simulink model "Progressive_Scan_Implementation_5x5_C"  (R2023a)
settings: Solver=VariableStepAuto  StartTime=0.0  StopTime=5  RelTol=1e-3
InitFcn:
  | Sampling_Time = 0.02;
  | 
  | % Find Controller
  | A_T= 3.6174;
  | tau = 1.2889;
  | Ts = Sampling_Time;
  | Kt = A_T * (1-exp(-Ts/tau));
  | poles = [-0.9180   -0.7439]; % 2x2
  | poles = [-0.5844   -0.9007]; % more aggressive
  | poles = [-0.7161   -0.8]; % 0.02 Ts aggro
  | poles = [-0.6161   -0.7]; % 0.02 Ts aggro
  | a1 = (poles(1)+poles(2)+1+exp(-Ts/tau))/Kt;
  | a0 = (poles(1)*poles(2)-exp(-Ts/tau))/Kt;
  | a1 = a1(1);
  | a0 = a0(1);
StopFcn:
  | datloc = out.varout{1}.Values;
  | 
  | t = datloc.Time;
  | T = datloc.Data;
  | writematrix([t T], "temp_out.csv");
  | cu = out.cuout{1}.Values;
  | writematrix([cu.Time cu.Data], "temp_control.csv");
settings Model: Creator=wangj  LastModifiedBy=wangj

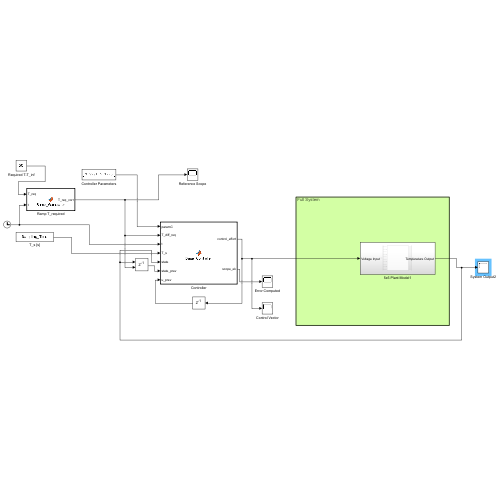
[thumbnail: Simulink's stored preview of the top-level diagram]
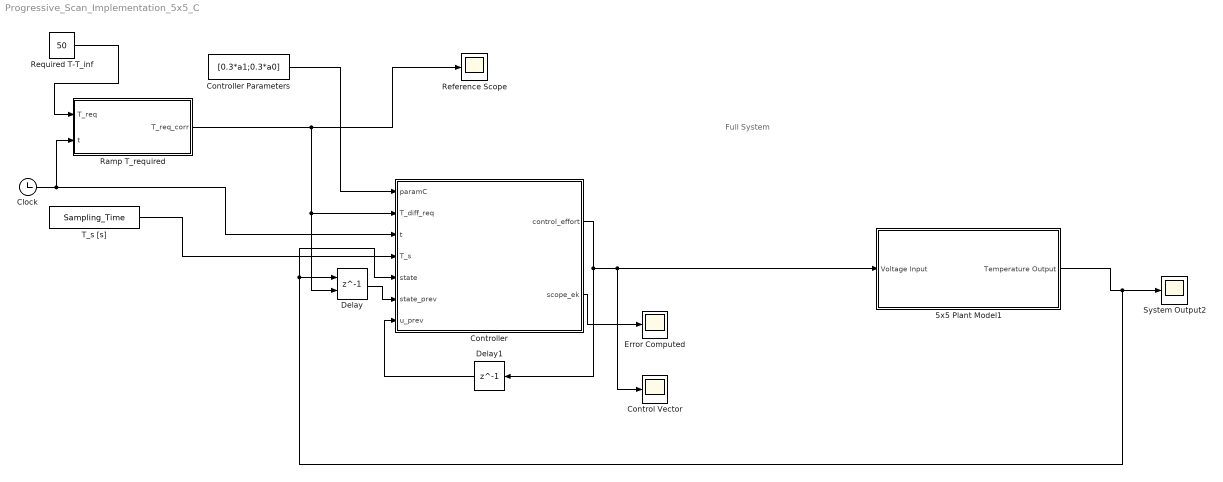
== system Progressive_Scan_Implementation_5x5_C ==
  note: Full System
  5x5 Plant Model1 : Subsystem
  Clock : Clock
  Control Vector : Scope
  Controller : MATLAB Function  TreatAsAtomicUnit=on
  Controller Parameters : Constant  Value=[0.3*a1;0.3*a0]
  Delay : Delay  DelayLength=1  InitialConditionSource=Input port
      settings: InputPortMap=u0,p4
  Delay1 : Delay  DelayLength=1
  Error Computed : Scope
  Ramp T_required : MATLAB Function  TreatAsAtomicUnit=on
  Reference Scope : Scope
  Required T-T_inf : Constant  Value=50
  System Output2 : Scope
  T_s [s] : Constant  Value=Sampling_Time
  wires:
  5x5 Plant Model1/1(Temperature Output) -> Controller/5(state), Delay/1, System Output2/1
  Delay/1 -> Controller/6(state_prev)
  Delay1/1 -> Controller/7(u_prev)
  Controller/1(control_effort) -> Delay1/1, 5x5 Plant Model1/1(Voltage Input), Control Vector/1
  Controller/2(scope_ek) -> Error Computed/1
  Ramp T_required/1(T_req_corr) -> Reference Scope/1, Delay/2, Controller/2(T_diff_req)
  Clock/1 -> Controller/3(t), Ramp T_required/2(t)
  T_s [s]/1 -> Controller/4(T_s)
  Controller Parameters/1 -> Controller/1(paramC)
  Required T-T_inf/1 -> Ramp T_required/1(T_req)

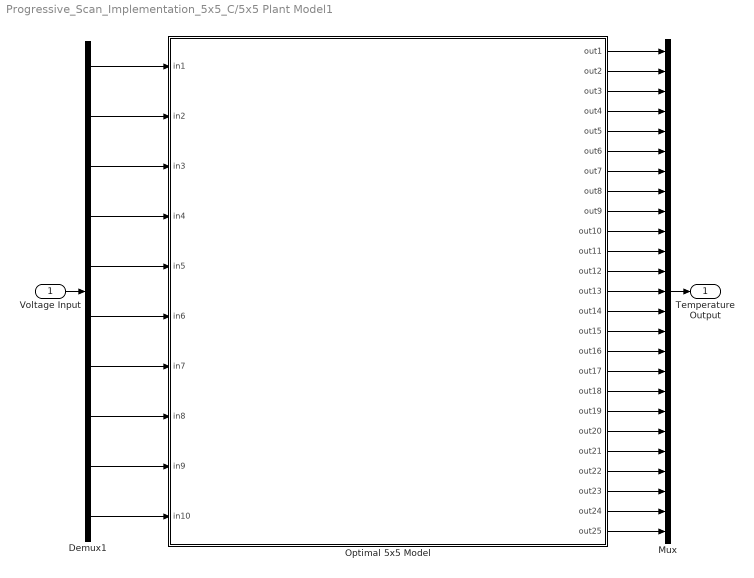
== system Progressive_Scan_Implementation_5x5_C/5x5 Plant Model1 ==
  Voltage Input : Inport
  Demux1 : Demux  Outputs=10
  Mux : Mux  Inputs=25
  Optimal 5x5 Model : Subsystem  mask(COMSOL Multiphysics Block){filename=D:\Dhiro_Files\Progressive Scan 5x5\5x5_optimal_77.fmu, dt=Ts}
      mask prompts: dt "Communication step size"
      mask help: COMSOL Multiphysics Block version 6.1
      mask init:
      | if exist('cosimblockinit')==0
      |    error('Can not initialize block. Start COMSOL with Simulink and try again')
      | else
      |     cosimblockinit
      | end
      mask DialogControl bp Prompt: Block Parameters
      mask DialogControl bp Callback: setblockparameters
      mask Display:
      | if isempty(filename)
      |     root = char(java.lang.System.getProperty('cs.root'));
      |     if ~isempty(root)
      |         filename = fullfile(root, 'ext\LiveLink\Simulink\resources\llsimulink_comsol_logo_256.bmp');
      |         if exist(filename, 'file')
      |             im = imread(filename);
      |         end
      |     end
      | end
      | if exist('im', 'var')
      |     image(im)
      | else
      |     disp('COMSOL')
      | end
      | 
      | if exist('labels', 'var')
      |     if isfield(labels, 'in')
      |         for i=1:length(labels.in)
      |             port_label('input', i, labels.in{i})
      |         end
      |     end
      | 
      |     if isfield(labels, 'out')
      |         for i=1:length(labels.out)
      |             port_label('output', i, labels.out{i})
      |         end
      |     end
      | end
  Temperature Output : Outport
  wires:
  Voltage Input/1 -> Demux1/1
  Optimal 5x5 Model/23(out23) -> Mux/23
  Optimal 5x5 Model/20(out20) -> Mux/20
  Optimal 5x5 Model/6(out6) -> Mux/6
  Optimal 5x5 Model/8(out8) -> Mux/8
  Demux1/2 -> Optimal 5x5 Model/2(in2)
  Optimal 5x5 Model/2(out2) -> Mux/2
  Optimal 5x5 Model/4(out4) -> Mux/4
  Demux1/1 -> Optimal 5x5 Model/1(in1)
  Optimal 5x5 Model/15(out15) -> Mux/15
  Optimal 5x5 Model/11(out11) -> Mux/11
  Optimal 5x5 Model/1(out1) -> Mux/1
  Optimal 5x5 Model/21(out21) -> Mux/21
  Optimal 5x5 Model/5(out5) -> Mux/5
  Optimal 5x5 Model/12(out12) -> Mux/12
  Optimal 5x5 Model/3(out3) -> Mux/3
  Optimal 5x5 Model/7(out7) -> Mux/7
  Optimal 5x5 Model/16(out16) -> Mux/16
  Optimal 5x5 Model/13(out13) -> Mux/13
  Optimal 5x5 Model/10(out10) -> Mux/10
  Demux1/3 -> Optimal 5x5 Model/3(in3)
  Optimal 5x5 Model/9(out9) -> Mux/9
  Optimal 5x5 Model/24(out24) -> Mux/24
  Optimal 5x5 Model/18(out18) -> Mux/18
  Demux1/5 -> Optimal 5x5 Model/5(in5)
  Optimal 5x5 Model/25(out25) -> Mux/25
  Optimal 5x5 Model/14(out14) -> Mux/14
  Optimal 5x5 Model/19(out19) -> Mux/19
  Optimal 5x5 Model/17(out17) -> Mux/17
  Optimal 5x5 Model/22(out22) -> Mux/22
  Demux1/7 -> Optimal 5x5 Model/7(in7)
  Demux1/8 -> Optimal 5x5 Model/8(in8)
  Demux1/9 -> Optimal 5x5 Model/9(in9)
  Mux/1 -> Temperature Output/1
  Demux1/10 -> Optimal 5x5 Model/10(in10)
  Demux1/6 -> Optimal 5x5 Model/6(in6)
  Demux1/4 -> Optimal 5x5 Model/4(in4)

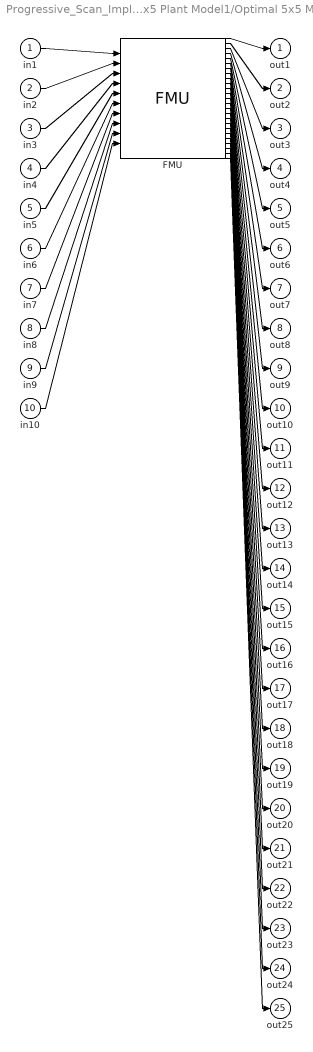
== system Progressive_Scan_Implementation_5x5_C/5x5 Plant Model1/Optimal 5x5 Model ==
  in1 : Inport
  in2 : Inport  Port=2
  in3 : Inport  Port=3
  in4 : Inport  Port=4
  in5 : Inport  Port=5
  in6 : Inport  Port=6
  in7 : Inport  Port=7
  in8 : Inport  Port=8
  in9 : Inport  Port=9
  in10 : Inport  Port=10
  FMU : FMU  FMUName=5x5_optimal_77.fmu  FMUDebugLogging=on  FMUMode=CoSimulation  FMUSampleTime=Ts
      mask Type: Optim_5x5.mph [Co-Simulation, v2.0]
      mask Display:
      | if (exist([Simulink.fileGenControl('get','CacheFolder') '\slprj\_fmu\8f427680cd09abf412d021646870dffe\5x5_optimal_77\model.png'],'file'))
      |     image([Simulink.fileGenControl('get','CacheFolder') '\slprj\_fmu\8f427680cd09abf412d021646870dffe\5x5_optimal_77\model.png']);
      | else
      |     disp('Optim_5x5.mph');
      | end
      | port_label('output',1,'comp1.m11(comp1.T)-293.15');
      | port_label('output',2,'comp1.m12(comp1.T)-293.15');
      | port_label('output',3,'comp1.m13(comp1.T)-293.15');
      | port_label('output',4,'comp1.m14(comp1.T)-293.15');
      | port_label('output',5,'comp1.m15(comp1.T)-293.15');
      | port_label('output',6,'comp1.m21(comp1.T)-293.15');
      | port_label('output',7,'comp1.m22(comp1.T)-293.15');
      | port_label('output',8,'comp1.m23(comp1.T)-293.15');
      | port_label('output',9,'comp1.m24(comp1.T)-293.15');
      | port_label('output',10,'comp1.m25(comp1.T)-293.15');
      | port_label('output',11,'comp1.m31(comp1.T)-293.15');
      | port_label('output',12,'comp1.m32(comp1.T)-293.15');
      | port_label('output',13,'comp1.m33(comp1.T)-293.15');
      | port_label('output',14,'comp1.m34(comp1.T)-293.15');
      | port_label('output',15,'comp1.m35(comp1.T)-293.15');
      | port_label('output',16,'comp1.m41(comp1.T)-293.15');
      | port_label('output',17,'comp1.m42(comp1.T)-293.15');
      | port_label('output',18,'comp1.m43(comp1.T)-293.15');
      | port_label('output',19,'comp1.m44(comp1.T)-293.15');
      | port_label('output',20,'comp1.m45(comp1.T)-293.15');
      | port_label('output',21,'comp1.m51(comp1.T)-293.15');
      | port_label('output',22,'comp1.m52(comp1.T)-293.15');
      | port_label('output',23,'comp1.m53(comp1.T)-293.15');
      | port_label('output',24,'comp1.m54(comp1.T)-293.15');
      | port_label('output',25,'comp1.m55(comp1.T)-293.15');
      | port_label('input',1,'X1');
      | port_label('input',2,'X2');
      | port_label('input',3,'X3');
      | port_label('input',4,'X4');
      | port_label('input',5,'X5');
      | port_label('input',6,'Y1');
      | port_label('input',7,'Y2');
      | port_label('input',8,'Y3');
      | port_label('input',9,'Y4');
      | port_label('input',10,'Y5');
  out1 : Outport
  out2 : Outport  Port=2
  out3 : Outport  Port=3
  out4 : Outport  Port=4
  out5 : Outport  Port=5
  out6 : Outport  Port=6
  out7 : Outport  Port=7
  out8 : Outport  Port=8
  out9 : Outport  Port=9
  out10 : Outport  Port=10
  out11 : Outport  Port=11
  out12 : Outport  Port=12
  out13 : Outport  Port=13
  out14 : Outport  Port=14
  out15 : Outport  Port=15
  out16 : Outport  Port=16
  out17 : Outport  Port=17
  out18 : Outport  Port=18
  out19 : Outport  Port=19
  out20 : Outport  Port=20
  out21 : Outport  Port=21
  out22 : Outport  Port=22
  out23 : Outport  Port=23
  out24 : Outport  Port=24
  out25 : Outport  Port=25
  wires:
  in1/1 -> FMU/1
  in2/1 -> FMU/2
  in3/1 -> FMU/3
  in4/1 -> FMU/4
  in5/1 -> FMU/5
  in6/1 -> FMU/6
  in7/1 -> FMU/7
  in8/1 -> FMU/8
  in9/1 -> FMU/9
  in10/1 -> FMU/10
  FMU/1 -> out1/1
  FMU/2 -> out2/1
  FMU/3 -> out3/1
  FMU/4 -> out4/1
  FMU/5 -> out5/1
  FMU/6 -> out6/1
  FMU/7 -> out7/1
  FMU/8 -> out8/1
  FMU/9 -> out9/1
  FMU/10 -> out10/1
  FMU/11 -> out11/1
  FMU/12 -> out12/1
  FMU/13 -> out13/1
  FMU/14 -> out14/1
  FMU/15 -> out15/1
  FMU/16 -> out16/1
  FMU/17 -> out17/1
  FMU/18 -> out18/1
  FMU/19 -> out19/1
  FMU/20 -> out20/1
  FMU/21 -> out21/1
  FMU/22 -> out22/1
  FMU/23 -> out23/1
  FMU/24 -> out24/1
  FMU/25 -> out25/1

== matlab function Progressive_Scan_Implementation_5x5_C/Controller ==
  data: paramC input; T_diff_req input; t input; T_s input; state input; state_prev input; u_prev input; control_effort output; scope_ek output
function [control_effort, scope_ek] = Base_Controller(paramC, T_diff_req, t, T_s, state, state_prev, u_prev)

% control_effort = zeros(4,1);
k = floor(t/T_s);

cn = mod(k,5)+1;

% % Well Shape Input
% input_filter_sel = [0 1 1 1 0 0 1 1 1 0;
%                     0 0.5 0.5 0.5 0.5, 0.5 0.5 0.5 0.5 1;
%                     0 0.5 0.5 0.5 0.5, 1 0.5 0.5 0.5 0.5;
%                     0.5 0.5 0.5 0.5 0, 1 0.5 0.5 0.5 0.5;
%                     0.5 0.5 0.5 0.5 0, 0.5 0.5 0.5 0.5 1;];
% 
% ref_vec_sel = [0 1 1 1 0 1 0 0 0 1 1 0 0 0 1 1 0 0 0 1 0 1 1 1 0;
%                0 0 0 0 1 0 0 0 0 0 0 0 0 0 0 0 0 0 0 0 0 0 0 0 0;
%                1 0 0 0 0 0 0 0 0 0 0 0 0 0 0 0 0 0 0 0 0 0 0 0 0;
%                0 0 0 0 0 0 0 0 0 0 0 0 0 0 0 0 0 0 0 0 1 0 0 0 0;
%                0 0 0 0 0 0 0 0 0 0 0 0 0 0 0 0 0 0 0 0 0 0 0 0 1];

% Cross Shape
% input_filter_sel = [0.5 1 0.5 0.5 0.5, 0.5 0.5 0.5 0 0.5;
%                     0.5 1 0.5 0.5 0.5, 0.5 0 0.5 0.5 0.5;
%                     0.5 0.5 1 0.5 0.5, 0.5 0.5 0 0.5 0.5;
%                     0.5 0.5 0.5 1 0.5, 0.5 0 0.5 0.5 0.5;
%                     0.5 0.5 0.5 1 0.5, 0.5 0.5 0.5 0 0.5;];
% 
% ref_vec_sel = [0 0 0 0 0, 0 0 0 1 0, 0 0 0 0 0, 0 0 0 0 0, 0 0 0 0 0;
%                0 0 0 0 0, 0 1 0 0 0, 0 0 0 0 0, 0 0 0 0 0, 0 0 0 0 0;
%                0 0 0 0 0, 0 0 0 0 0, 0 0 1 0 0, 0 0 0 0 0, 0 0 0 0 0;
%                0 0 0 0 0, 0 0 0 0 0, 0 0 0 0 0, 0 1 0 0 0, 0 0 0 0 0;
%                0 0 0 0 0, 0 0 0 0 0, 0 0 0 0 0, 0 0 0 1 0, 0 0 0 0 0];

% Diag Shape
input_filter_sel = [1 0.5 0.5 0.5 0.5, 0 0.5 0.5 0.5 0.5;
                    0.5 1 0.5 0.5 0.5, 0.5 0 0.5 0.5 0.5;
                    0.5 0.5 1 0.5 0.5, 0.5 0.5 0 0.5 0.5;
                    0.5 0.5 0.5 1 0.5, 0.5 0.5 0.5 0 0.5;
                    0.5 0.5 0.5 0.5 1, 0.5 0.5 0.5 0.5 0;];

ref_vec_sel = [1 0 0 0 0, 0 0 0 0 0, 0 0 0 0 0, 0 0 0 0 0, 0 0 0 0 0;
               0 0 0 0 0, 0 1 0 0 0, 0 0 0 0 0, 0 0 0 0 0, 0 0 0 0 0;
               0 0 0 0 0, 0 0 0 0 0, 0 0 1 0 0, 0 0 0 0 0, 0 0 0 0 0;
               0 0 0 0 0, 0 0 0 0 0, 0 0 0 0 0, 0 0 0 1 0, 0 0 0 0 0;
               0 0 0 0 0, 0 0 0 0 0, 0 0 0 0 0, 0 0 0 0 0, 0 0 0 0 1];



input_filter = input_filter_sel(cn, :).';

ref_req = T_diff_req; % activation state
ref_vec = ref_vec_sel(cn, :).';
e_k = - max(ref_vec.*state) + ref_req;
e_k_prev = - max(ref_vec.*state_prev) + ref_req;

a1 = paramC(1); a0 = paramC(2);
apf = find(input_filter==1);

cf = u_prev(apf(1)) + a1 * e_k + a0 * e_k_prev;

if cf < 0
    cf = 0;
end

% control_effort = sqrt(cf) * input_filter;
control_effort = cf * input_filter;
scope_ek = control_effort;
end

== matlab function Progressive_Scan_Implementation_5x5_C/Ramp T_required ==
  data: T_req input; T_req_corr output; t input
function T_req_corr = Ramp_Generator(T_req, t)

tT = 2;

T_req_corr = (T_req/tT)*t;
if t >= tT
    T_req_corr = T_req;
end

end
